simulink model "Motor_Satellite_Dynamics"  (R2024b)
settings: Solver=VariableStepAuto  StartTime=0.0  StopTime=10.0  RelTol=1e-3
undefined symbols (not defined in the file or in its folder): J_rotor, J_satelit
settings Model: Creator=bbtp  LastModifiedBy=bbtp

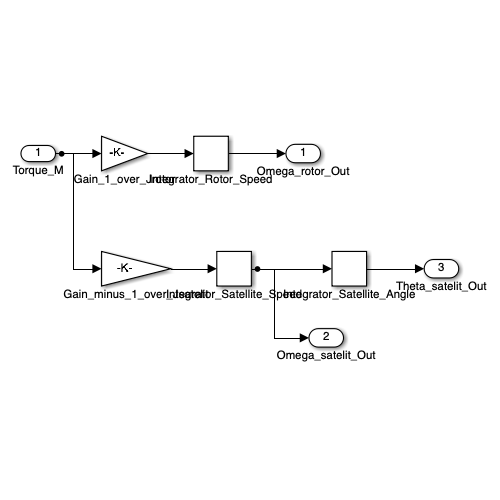
[thumbnail: Simulink's stored preview of the top-level diagram]
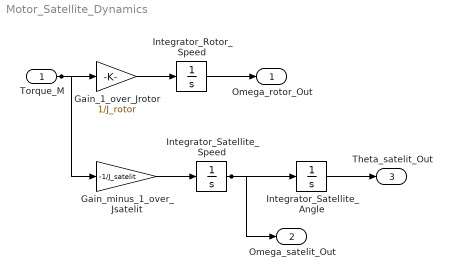
== system Motor_Satellite_Dynamics ==
  Torque_M : Inport
  Gain_1_over_Jrotor : Gain  Gain=1/J_rotor
  Gain_minus_1_over_Jsatelit : Gain  Gain=-1/J_satelit
  Integrator_Rotor_Speed : Integrator
  Integrator_Satellite_Angle : Integrator
  Integrator_Satellite_Speed : Integrator
  Omega_rotor_Out : Outport
  Omega_satelit_Out : Outport  Port=2
  Theta_satelit_Out : Outport  Port=3
  wires:
  Torque_M/1 -> Gain_1_over_Jrotor/1, Gain_minus_1_over_Jsatelit/1
  Gain_1_over_Jrotor/1 -> Integrator_Rotor_Speed/1
  Integrator_Rotor_Speed/1 -> Omega_rotor_Out/1
  Gain_minus_1_over_Jsatelit/1 -> Integrator_Satellite_Speed/1
  Integrator_Satellite_Speed/1 -> Integrator_Satellite_Angle/1, Omega_satelit_Out/1
  Integrator_Satellite_Angle/1 -> Theta_satelit_Out/1
